simulink model "StewartDynamics"  (R2015a)
settings: Solver=ode45  StartTime=0.0  StopTime=10.0  RelTol=1e-3
undefined symbols (not defined in the file or in its folder): body_pts
libraries: simulink x1
settings Model: Creator=admin  LastModifiedBy=admin

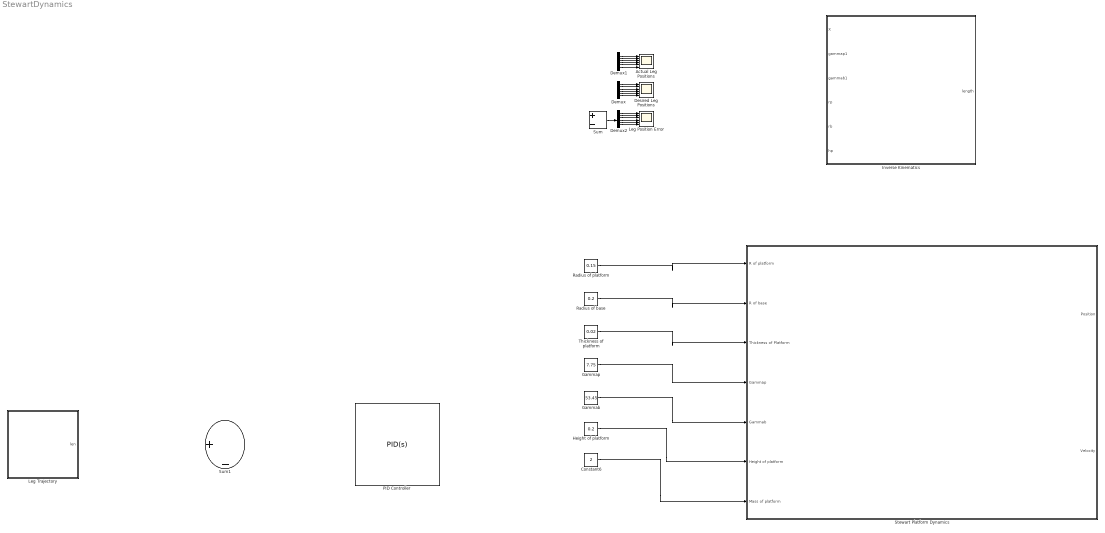
== system StewartDynamics ==
  Actual Leg Positions : Scope  NumInputPorts=6
      settings: TimeRange=10  YMin=0~1~0~0~0~0  YMax=14~14~13~14~13~13  SaveName=ScopeData5
  Constant6 : Constant  Value=2
  Demux : Demux  Outputs=6
  Demux1 : Demux  Outputs=6
  Demux2 : Demux  Outputs=6
  Desired Leg Positions : Scope  NumInputPorts=6
      settings: YMin=0~0~0~0~0~0  YMax=15~15~13~13~14~14  SaveName=ScopeData4
  Gammab : Constant  Value=53.45
  Gammap : Constant  Value=7.75
  Height of platform : Constant  Value=0.2
  Inverse Kinematics : MATLAB Function  TreatAsAtomicUnit=on
  Leg Trajectory : Subsystem
  Leg Position Error : Scope  NumInputPorts=6
      settings: YMin=-0.2~-0.2~-0.2~-0.2~-0.2~-0.2  YMax=0.2~0.2~0.2~0.2~0.2~0.2  SaveName=ScopeData6
  PID Controller : simulink/Continuous/PID Controller  Controller=PID  TimeDomain=Continuous-time  SampleTime=-1  IntegratorMethod=Forward Euler  FilterMethod=Forward Euler  Form=Parallel  UseFilter=on  ControllerParametersSource=internal  P=1  I=1  D=0  N=100  InitialConditionSource=internal  InitialConditionForIntegrator=0  InitialConditionForFilter=0  ExternalReset=none  LimitOutput=off  UpperSaturationLimit=inf  LowerSaturationLimit=-inf  LinearizeAsGain=on  AntiWindupMode=none  Kb=1  TrackingMode=off  Kt=1  PParamMin=[]  PParamMax=[]  IParamMin=[]  IParamMax=[]  DParamMin=[]  DParamMax=[]  NParamMin=[]  NParamMax=[]  KbParamMin=[]  KbParamMax=[]  KtParamMin=[]  KtParamMax=[]  POutMin=[]  POutMax=[]  IOutMin=[]  IOutMax=[]  DOutMin=[]  DOutMax=[]  NOutMin=[]  NOutMax=[]  KbOutMin=[]  KbOutMax=[]  KtOutMin=[]  KtOutMax=[]  IntegratorOutMin=[]  IntegratorOutMax=[]  FilterOutMin=[]  FilterOutMax=[]  SumOutMin=[]  SumOutMax=[]  SumI1OutMin=[]  SumI1OutMax=[]  SumI2OutMin=[]  SumI2OutMax=[]  SumI3OutMin=[]  SumI3OutMax=[]  SumDOutMin=[]  SumDOutMax=[]  SaturationOutMin=[]  SaturationOutMax=[]  IntegratorContinuousStateAttributes=''  IntegratorStateMustResolveToSignalObject=off  IntegratorRTWStateStorageClass=Auto  FilterContinuousStateAttributes=''  FilterStateMustResolveToSignalObject=off  FilterRTWStateStorageClass=Auto  DifferentiatorICPrevScaledInput=0  DifferentiatorOutMin=[]  DifferentiatorOutMax=[]
  Radius of base : Constant  Value=0.2
  Radius of platform : Constant  Value=0.15
  Stewart Platform Dynamics : Subsystem
  Sum : Sum  Inputs=+-
  Sum1 : Sum  Inputs=|+-
  Thickness of platform : Constant  Value=0.02
  wires:
  Gammap/1 -> Stewart Platform Dynamics/4(Gammap)
  Gammab/1 -> Stewart Platform Dynamics/5(Gammab)
  Height of platform/1 -> Stewart Platform Dynamics/6("Height of platform ")
  Constant6/1 -> Stewart Platform Dynamics/7(Mass of platform)
  Demux/1 -> Desired Leg Positions/1
  Demux/2 -> Desired Leg Positions/2
  Demux/3 -> Desired Leg Positions/3
  Demux/4 -> Desired Leg Positions/4
  Demux/5 -> Desired Leg Positions/5
  Demux/6 -> Desired Leg Positions/6
  Demux1/1 -> Actual Leg Positions/1
  Demux1/2 -> Actual Leg Positions/2
  Demux1/3 -> Actual Leg Positions/3
  Demux1/4 -> Actual Leg Positions/4
  Demux1/5 -> Actual Leg Positions/5
  Demux1/6 -> Actual Leg Positions/6
  Demux2/1 -> Leg Position Error/1
  Demux2/2 -> Leg Position Error/2
  Demux2/3 -> Leg Position Error/3
  Demux2/4 -> Leg Position Error/4
  Demux2/5 -> Leg Position Error/5
  Demux2/6 -> Leg Position Error/6
  Sum/1 -> Demux2/1
  Radius of platform/1 -> Stewart Platform Dynamics/1(R of platform)
  Radius of base/1 -> Stewart Platform Dynamics/2(R of base)
  Thickness of platform/1 -> Stewart Platform Dynamics/3(Thickness of Platform)
  ? -> ?
  ? -> ?
  ? -> ?
  ? -> ?

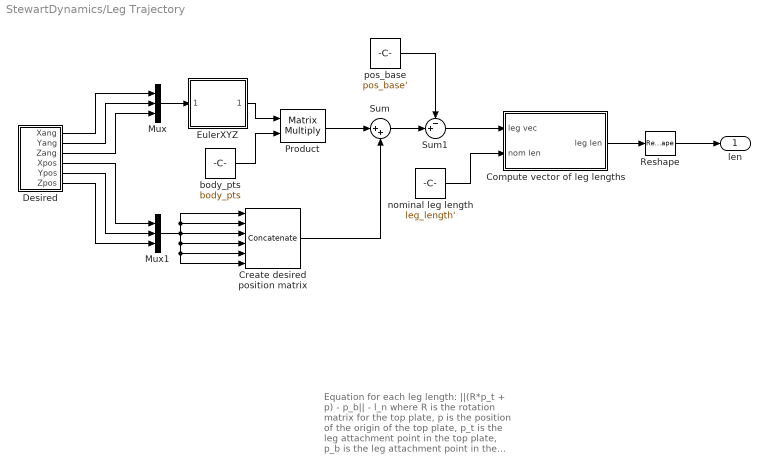
== system StewartDynamics/Leg Trajectory ==
  note: Equation for each leg length:
      | ||(R*p_t + p) - p_b|| - l_n
      | where R is the rotation matrix
      | for the top plate, p is the position
      | of the origin of the top plate, p_t
      | is the leg attachment point in the
      | top plate, p_b is the leg attachment
      | point in the base, and l_n is the
      | nominal distance between the
      | top and base attachment points.
  Compute vector of leg lengths : Subsystem  TreatAsAtomicUnit=on
  Create desired position matrix : Concatenate  NumInputs=6  Mode=Multidimensional array  ConcatenateDimension=2
  Desired : Subsystem
  EulerXYZ : Subsystem  AncestorBlock=|  mask(EulerXYZ){}
      | aerospace/Axes
      | Transformations/Direction Cosine Matrix
      | from Euler Angles
      mask help: Creates the EulerXYZ rotation matrix corresponding to body fixed rotations in the X, Y, and then Z. This matrix maps body vectors to world vectors.
      mask Help:
      | <p>This block determines the EulerXYZ matrix from a 3x1 euler angles in the X, Y, & Z directions. The matrix maps vectors the body axes to the inertial axes.</p>
      | 
      | <p>The block input and output contain more than one signal as described below.</p>
      | 
      | <p><H4>Block Vector Input - Euler XYZ angles</H4>
      |     <ul>
      |     <li>X angle</li>
      |     <li>Y angle</li>
      |     <li>Z angle</li>
      |    </ul>
      |    </p>
      | 
      | <p><H4>Block Matrix Output - XYZ Euler Matrix </H4>
      |     <ul>
      |    </ul>
      |    </p>
      mask Display: disp('Rotation\nMatrix')
  Mux : Mux  Inputs=3
  Mux1 : Mux  Inputs=3
  Product : Product  Multiplication=Matrix(*)  SaturateOnIntegerOverflow=on  InputSameDT=on  OutDataTypeStr=Inherit: Same as first input
  Reshape : Reshape
  Sum : Sum  Inputs=|++  SaturateOnIntegerOverflow=on  InputSameDT=on  OutDataTypeStr=Inherit: Same as first input
  Sum1 : Sum  Inputs=-+|  SaturateOnIntegerOverflow=on  InputSameDT=on  OutDataTypeStr=Inherit: Same as first input
  body_pts : Constant  Value=body_pts  VectorParams1D=off
  nominal leg length : Constant  Value=leg_length'  VectorParams1D=off
  pos_base : Constant  Value=pos_base'  VectorParams1D=off
  len : Outport
  wires:
  Mux/1 -> EulerXYZ/1(x y z angles)
  EulerXYZ/1(EulerXYZ) -> Product/1
  body_pts/1 -> Product/2
  Product/1 -> Sum/1
  Mux1/1 -> Create desired position matrix/1, Create desired position matrix/2, Create desired position matrix/4, Create desired position matrix/5, Create desired position matrix/6, Create desired position matrix/3
  Create desired position matrix/1 -> Sum/2
  pos_base/1 -> Sum1/1
  Sum/1 -> Sum1/2
  Sum1/1 -> Compute vector of leg lengths/1(leg vec)
  nominal leg length/1 -> Compute vector of leg lengths/2(nom len)
  Compute vector of leg lengths/1(leg len) -> Reshape/1
  Desired/3(Zang) -> Mux/3
  Desired/1(Xang) -> Mux/1
  Desired/2(Yang) -> Mux/2
  Desired/4(Xpos) -> Mux1/1
  Desired/5(Ypos) -> Mux1/2
  Desired/6(Zpos) -> Mux1/3
  Reshape/1 -> len/1

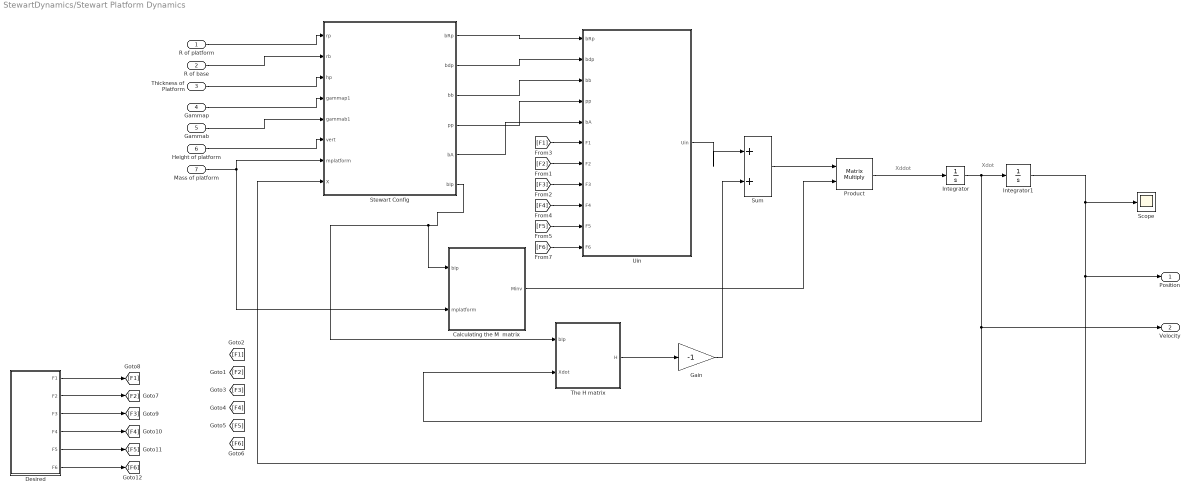
== system StewartDynamics/Stewart Platform Dynamics ==
  note: Xdot
  note: Xddot
  R of platform : Inport
  R of base : Inport  Port=2
  Thickness of Platform : Inport  Port=3
  Gammap : Inport  Port=4
  Gammab : Inport  Port=5
  "Height of platform " : Inport  Port=6
  Mass of platform : Inport  Port=7
  Calculating the M  matrix : MATLAB Function  TreatAsAtomicUnit=on
  Desired : Subsystem
  Gain : Gain  Gain=-1
  Integrator : Integrator
  Integrator1 : Integrator
  Product : Product  Multiplication=Matrix(*)
  Scope : Scope
  Stewart Config : MATLAB Function  TreatAsAtomicUnit=on
  Sum : Sum  Inputs=|++
  The H matrix : MATLAB Function  TreatAsAtomicUnit=on
  Uin : MATLAB Function  TreatAsAtomicUnit=on
  Position : Outport
  Velocity : Outport  Port=2
  wires:
  R of platform/1 -> Stewart Config/1(rp)
  "Height of platform "/1 -> Stewart Config/6(vert)
  Gammap/1 -> Stewart Config/4(gammap1)
  Gammab/1 -> Stewart Config/5(gammab1)
  Thickness of Platform/1 -> Stewart Config/3(hp)
  Mass of platform/1 -> Calculating the M  matrix/2(mplatform), Stewart Config/7(mplatform)
  R of base/1 -> Stewart Config/2(rb)
  Stewart Config/6(bIp) -> Calculating the M  matrix/1(bIp), The H matrix/1(bIp)
  Stewart Config/5(bA) -> Uin/5(bA)
  Stewart Config/4(pp) -> Uin/4(pp)
  Integrator1/1 -> Scope/1, Position/1, Stewart Config/8(X)
  Integrator/1 -> Integrator1/1, Velocity/1, The H matrix/2(Xdot)
  Product/1 -> Integrator/1
  The H matrix/1(H) -> Gain/1
  Stewart Config/1(bRp) -> Uin/1(bRp)
  Calculating the M  matrix/1(Minv) -> Product/2
  Sum/1 -> Product/1
  Stewart Config/3(bb) -> Uin/3(bb)
  Uin/1(Uin) -> Sum/1
  Stewart Config/2(bdp) -> Uin/2(bdp)
  Gain/1 -> Sum/2
  ? -> [F1]
  ? -> [F2]
  ? -> [F3]
  ? -> [F4]
  ? -> [F5]
  ? -> [F6]
  [F1] -> Uin/6(F1)
  [F2] -> Uin/7(F2)
  [F3] -> Uin/8(F3)
  [F4] -> Uin/9(F4)
  [F5] -> Uin/10(F5)
  [F6] -> Uin/11(F6)
  Desired/1(F1) -> [F1]
  Desired/2(F2) -> [F2]
  Desired/3(F3) -> [F3]
  Desired/4(F4) -> [F4]
  Desired/5(F5) -> [F5]
  Desired/6(F6) -> [F6]

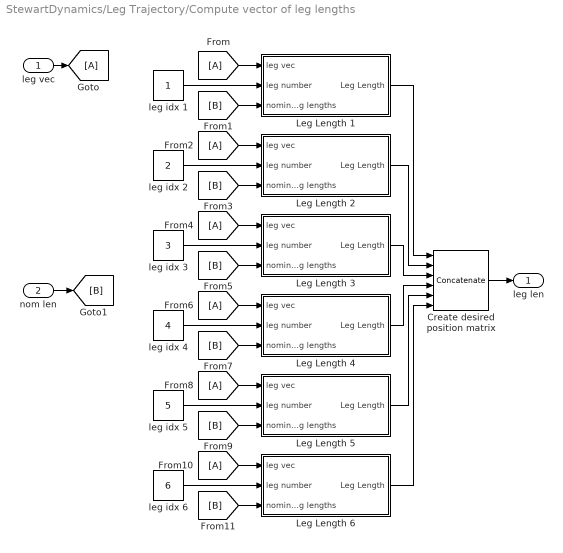
== system StewartDynamics/Leg Trajectory/Compute vector of leg lengths ==
  leg vec : Inport
  nom len : Inport  Port=2
  Create desired position matrix : Concatenate  NumInputs=6  Mode=Multidimensional array  ConcatenateDimension=2
  Leg Length 1 : Subsystem
  Leg Length 2 : Subsystem
  Leg Length 3 : Subsystem
  Leg Length 4 : Subsystem
  Leg Length 5 : Subsystem
  Leg Length 6 : Subsystem
  leg idx 1 : Constant
  leg idx 2 : Constant  Value=2
  leg idx 3 : Constant  Value=3
  leg idx 4 : Constant  Value=4
  leg idx 5 : Constant  Value=5
  leg idx 6 : Constant  Value=6
  leg len : Outport
  wires:
  Leg Length 6/1(Leg Length) -> Create desired position matrix/6
  Leg Length 5/1(Leg Length) -> Create desired position matrix/5
  Leg Length 4/1(Leg Length) -> Create desired position matrix/4
  Leg Length 3/1(Leg Length) -> Create desired position matrix/3
  Leg Length 2/1(Leg Length) -> Create desired position matrix/2
  Leg Length 1/1(Leg Length) -> Create desired position matrix/1
  [B] -> Leg Length 6/3(nominal leg lengths)
  [A] -> Leg Length 6/1(leg vec)
  leg idx 6/1 -> Leg Length 6/2(leg number)
  [B] -> Leg Length 5/3(nominal leg lengths)
  [A] -> Leg Length 5/1(leg vec)
  leg idx 5/1 -> Leg Length 5/2(leg number)
  [B] -> Leg Length 4/3(nominal leg lengths)
  [A] -> Leg Length 4/1(leg vec)
  leg idx 4/1 -> Leg Length 4/2(leg number)
  [B] -> Leg Length 3/3(nominal leg lengths)
  [A] -> Leg Length 3/1(leg vec)
  leg idx 3/1 -> Leg Length 3/2(leg number)
  [B] -> Leg Length 2/3(nominal leg lengths)
  [A] -> Leg Length 2/1(leg vec)
  leg idx 2/1 -> Leg Length 2/2(leg number)
  [B] -> Leg Length 1/3(nominal leg lengths)
  nom len/1 -> [B]
  [A] -> Leg Length 1/1(leg vec)
  leg vec/1 -> [A]
  leg idx 1/1 -> Leg Length 1/2(leg number)
  Create desired position matrix/1 -> leg len/1

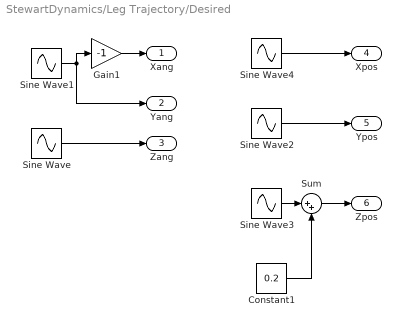
== system StewartDynamics/Leg Trajectory/Desired ==
  Constant1 : Constant  Value=0.2
  Gain1 : Gain  Gain=-1  SaturateOnIntegerOverflow=on  OutDataTypeStr=Inherit: Same as input  ParamDataTypeStr=Inherit: Same as input
  Sine Wave : Sin  Amplitude=0.03  Frequency=3  SampleTime=0
  Sine Wave1 : Sin  Amplitude=0.03  Frequency=3  SampleTime=0
  Sine Wave2 : Sin  Amplitude=0.025  Frequency=3  Phase=pi/2  SampleTime=0
  Sine Wave3 : Sin  Amplitude=0.025  Frequency=3  SampleTime=0
  Sine Wave4 : Sin  Amplitude=0.035  Frequency=3  SampleTime=0
  Sum : Sum  Inputs=|++  SaturateOnIntegerOverflow=on  InputSameDT=on  OutDataTypeStr=Inherit: Same as first input
  Xang : Outport
  Yang : Outport  Port=2
  Zang : Outport  Port=3
  Xpos : Outport  Port=4
  Ypos : Outport  Port=5
  Zpos : Outport  Port=6
  wires:
  Sine Wave/1 -> Zang/1
  Sine Wave1/1 -> Yang/1, Gain1/1
  Gain1/1 -> Xang/1
  Sine Wave2/1 -> Ypos/1
  Sine Wave3/1 -> Sum/1
  Sum/1 -> Zpos/1
  Constant1/1 -> Sum/2
  Sine Wave4/1 -> Xpos/1

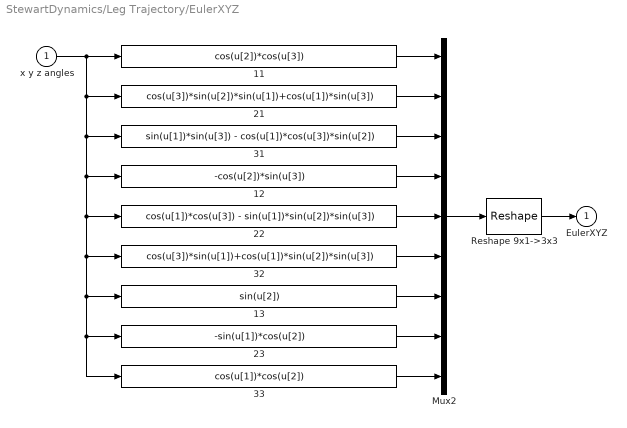
== system StewartDynamics/Leg Trajectory/EulerXYZ ==
  x y z angles : Inport
  11 : Fcn  Expr=cos(u[2])*cos(u[3])
  12 : Fcn  Expr=-cos(u[2])*sin(u[3])
  13 : Fcn  Expr=sin(u[2])
  21 : Fcn  Expr=cos(u[3])*sin(u[2])*sin(u[1])+cos(u[1])*sin(u[3])
  22 : Fcn  Expr=cos(u[1])*cos(u[3]) - sin(u[1])*sin(u[2])*sin(u[3])
  23 : Fcn  Expr=-sin(u[1])*cos(u[2])
  31 : Fcn  Expr=sin(u[1])*sin(u[3]) - cos(u[1])*cos(u[3])*sin(u[2])
  32 : Fcn  Expr=cos(u[3])*sin(u[1])+cos(u[1])*sin(u[2])*sin(u[3])
  33 : Fcn  Expr=cos(u[1])*cos(u[2])
  Mux2 : Mux  Inputs=9
  Reshape 9x1->3x3 : Reshape  OutputDimensionality=Customize  OutputDimensions=[3,3]
  EulerXYZ : Outport  InitialOutput=0
  wires:
  x y z angles/1 -> 23/1, 33/1, 13/1, 32/1, 22/1, 12/1, 31/1, 21/1, 11/1
  33/1 -> Mux2/9
  23/1 -> Mux2/8
  13/1 -> Mux2/7
  32/1 -> Mux2/6
  22/1 -> Mux2/5
  12/1 -> Mux2/4
  31/1 -> Mux2/3
  21/1 -> Mux2/2
  11/1 -> Mux2/1
  Mux2/1 -> Reshape 9x1->3x3/1
  Reshape 9x1->3x3/1 -> EulerXYZ/1

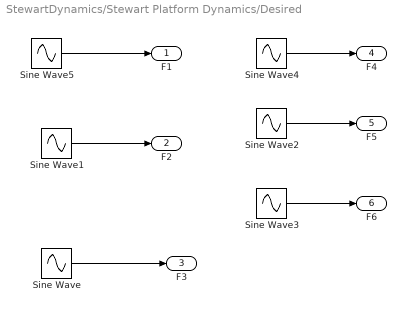
== system StewartDynamics/Stewart Platform Dynamics/Desired ==
  Sine Wave : Sin  Amplitude=0.29  Frequency=0.6283  SampleTime=0
  Sine Wave1 : Sin  Amplitude=0.3  Frequency=0.628  Phase=1.57  SampleTime=0
  Sine Wave2 : Sin  Amplitude=0.305  Frequency=0.6283  SampleTime=0
  Sine Wave3 : Sin  Amplitude=0.28  Frequency=0.6283  Phase=1.57  SampleTime=0
  Sine Wave4 : Sin  Amplitude=0.31  Frequency=0.6283  Phase=1.57  SampleTime=0
  Sine Wave5 : Sin  Amplitude=0.3  Frequency=0.628  SampleTime=0
  F1 : Outport
  F2 : Outport  Port=2
  F3 : Outport  Port=3
  F4 : Outport  Port=4
  F5 : Outport  Port=5
  F6 : Outport  Port=6
  wires:
  Sine Wave/1 -> F3/1
  Sine Wave1/1 -> F2/1
  Sine Wave5/1 -> F1/1
  Sine Wave2/1 -> F5/1
  Sine Wave3/1 -> F6/1
  Sine Wave4/1 -> F4/1

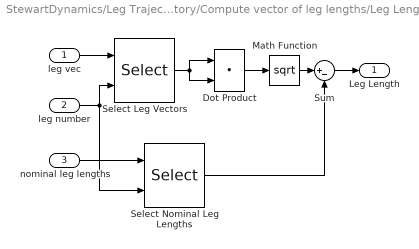
== system StewartDynamics/Leg Trajectory/Compute vector of leg lengths/Leg Length 1 ==
  leg vec : Inport
  leg number : Inport  Port=2
  nominal leg lengths : Inport  Port=3
  Dot Product : DotProduct  InputSameDT=on  OutDataTypeStr=Inherit: Inherit via internal rule
  Math Function : Math  Operator=sqrt  SaturateOnIntegerOverflow=on
  Select Leg Vectors : Selector  NumberOfDimensions=2  InputPortWidth=3  IndexOptions=Select all,Index vector (port)  Indices=-1,1
  Select Nominal Leg Lengths : Selector  InputPortWidth=6  IndexOptions=Index vector (port)  Indices=[1 3]
  Sum : Sum  Inputs=|+-  SaturateOnIntegerOverflow=on  InputSameDT=on  OutDataTypeStr=Inherit: Same as first input
  Leg Length : Outport
  wires:
  nominal leg lengths/1 -> Select Nominal Leg Lengths/1
  Sum/1 -> Leg Length/1
  leg vec/1 -> Select Leg Vectors/1
  leg number/1 -> Select Leg Vectors/2, Select Nominal Leg Lengths/2
  Dot Product/1 -> Math Function/1
  Select Leg Vectors/1 -> Dot Product/1, Dot Product/2
  Math Function/1 -> Sum/1
  Select Nominal Leg Lengths/1 -> Sum/2

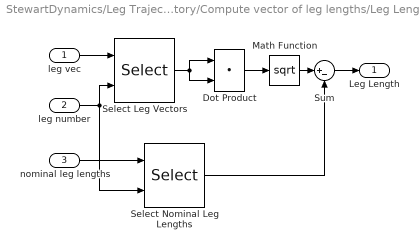
== system StewartDynamics/Leg Trajectory/Compute vector of leg lengths/Leg Length 2 ==
  leg vec : Inport
  leg number : Inport  Port=2
  nominal leg lengths : Inport  Port=3
  Dot Product : DotProduct  InputSameDT=on  OutDataTypeStr=Inherit: Inherit via internal rule
  Math Function : Math  Operator=sqrt  SaturateOnIntegerOverflow=on
  Select Leg Vectors : Selector  NumberOfDimensions=2  InputPortWidth=3  IndexOptions=Select all,Index vector (port)  Indices=-1,1
  Select Nominal Leg Lengths : Selector  InputPortWidth=6  IndexOptions=Index vector (port)  Indices=[1 3]
  Sum : Sum  Inputs=|+-  SaturateOnIntegerOverflow=on  InputSameDT=on  OutDataTypeStr=Inherit: Same as first input
  Leg Length : Outport
  wires:
  nominal leg lengths/1 -> Select Nominal Leg Lengths/1
  Sum/1 -> Leg Length/1
  leg vec/1 -> Select Leg Vectors/1
  leg number/1 -> Select Leg Vectors/2, Select Nominal Leg Lengths/2
  Dot Product/1 -> Math Function/1
  Select Leg Vectors/1 -> Dot Product/1, Dot Product/2
  Math Function/1 -> Sum/1
  Select Nominal Leg Lengths/1 -> Sum/2

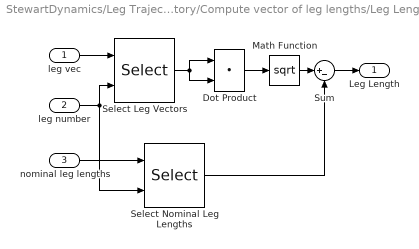
== system StewartDynamics/Leg Trajectory/Compute vector of leg lengths/Leg Length 3 ==
  leg vec : Inport
  leg number : Inport  Port=2
  nominal leg lengths : Inport  Port=3
  Dot Product : DotProduct  InputSameDT=on  OutDataTypeStr=Inherit: Inherit via internal rule
  Math Function : Math  Operator=sqrt  SaturateOnIntegerOverflow=on
  Select Leg Vectors : Selector  NumberOfDimensions=2  InputPortWidth=3  IndexOptions=Select all,Index vector (port)  Indices=-1,1
  Select Nominal Leg Lengths : Selector  InputPortWidth=6  IndexOptions=Index vector (port)  Indices=[1 3]
  Sum : Sum  Inputs=|+-  SaturateOnIntegerOverflow=on  InputSameDT=on  OutDataTypeStr=Inherit: Same as first input
  Leg Length : Outport
  wires:
  nominal leg lengths/1 -> Select Nominal Leg Lengths/1
  Sum/1 -> Leg Length/1
  leg vec/1 -> Select Leg Vectors/1
  leg number/1 -> Select Leg Vectors/2, Select Nominal Leg Lengths/2
  Dot Product/1 -> Math Function/1
  Select Leg Vectors/1 -> Dot Product/1, Dot Product/2
  Math Function/1 -> Sum/1
  Select Nominal Leg Lengths/1 -> Sum/2

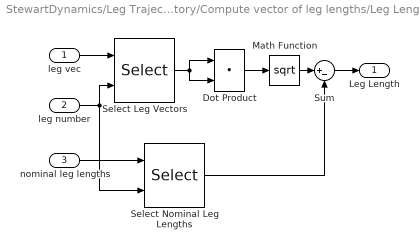
== system StewartDynamics/Leg Trajectory/Compute vector of leg lengths/Leg Length 4 ==
  leg vec : Inport
  leg number : Inport  Port=2
  nominal leg lengths : Inport  Port=3
  Dot Product : DotProduct  InputSameDT=on  OutDataTypeStr=Inherit: Inherit via internal rule
  Math Function : Math  Operator=sqrt  SaturateOnIntegerOverflow=on
  Select Leg Vectors : Selector  NumberOfDimensions=2  InputPortWidth=3  IndexOptions=Select all,Index vector (port)  Indices=-1,1
  Select Nominal Leg Lengths : Selector  InputPortWidth=6  IndexOptions=Index vector (port)  Indices=[1 3]
  Sum : Sum  Inputs=|+-  SaturateOnIntegerOverflow=on  InputSameDT=on  OutDataTypeStr=Inherit: Same as first input
  Leg Length : Outport
  wires:
  nominal leg lengths/1 -> Select Nominal Leg Lengths/1
  Sum/1 -> Leg Length/1
  leg vec/1 -> Select Leg Vectors/1
  leg number/1 -> Select Leg Vectors/2, Select Nominal Leg Lengths/2
  Dot Product/1 -> Math Function/1
  Select Leg Vectors/1 -> Dot Product/1, Dot Product/2
  Math Function/1 -> Sum/1
  Select Nominal Leg Lengths/1 -> Sum/2

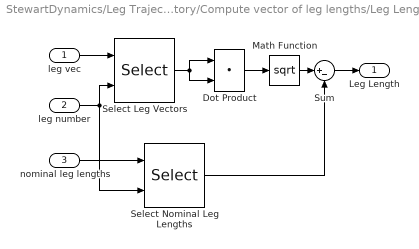
== system StewartDynamics/Leg Trajectory/Compute vector of leg lengths/Leg Length 5 ==
  leg vec : Inport
  leg number : Inport  Port=2
  nominal leg lengths : Inport  Port=3
  Dot Product : DotProduct  InputSameDT=on  OutDataTypeStr=Inherit: Inherit via internal rule
  Math Function : Math  Operator=sqrt  SaturateOnIntegerOverflow=on
  Select Leg Vectors : Selector  NumberOfDimensions=2  InputPortWidth=3  IndexOptions=Select all,Index vector (port)  Indices=-1,1
  Select Nominal Leg Lengths : Selector  InputPortWidth=6  IndexOptions=Index vector (port)  Indices=[1 3]
  Sum : Sum  Inputs=|+-  SaturateOnIntegerOverflow=on  InputSameDT=on  OutDataTypeStr=Inherit: Same as first input
  Leg Length : Outport
  wires:
  nominal leg lengths/1 -> Select Nominal Leg Lengths/1
  Sum/1 -> Leg Length/1
  leg vec/1 -> Select Leg Vectors/1
  leg number/1 -> Select Leg Vectors/2, Select Nominal Leg Lengths/2
  Dot Product/1 -> Math Function/1
  Select Leg Vectors/1 -> Dot Product/1, Dot Product/2
  Math Function/1 -> Sum/1
  Select Nominal Leg Lengths/1 -> Sum/2

== system StewartDynamics/Leg Trajectory/Compute vector of leg lengths/Leg Length 6 ==
  leg vec : Inport
  leg number : Inport  Port=2
  nominal leg lengths : Inport  Port=3
  Dot Product : DotProduct  InputSameDT=on  OutDataTypeStr=Inherit: Inherit via internal rule
  Math Function : Math  Operator=sqrt  SaturateOnIntegerOverflow=on
  Select Leg Vectors : Selector  NumberOfDimensions=2  InputPortWidth=3  IndexOptions=Select all,Index vector (port)  Indices=-1,1
  Select Nominal Leg Lengths : Selector  InputPortWidth=6  IndexOptions=Index vector (port)  Indices=[1 3]
  Sum : Sum  Inputs=|+-  SaturateOnIntegerOverflow=on  InputSameDT=on  OutDataTypeStr=Inherit: Same as first input
  Leg Length : Outport
  wires:
  nominal leg lengths/1 -> Select Nominal Leg Lengths/1
  Sum/1 -> Leg Length/1
  leg vec/1 -> Select Leg Vectors/1
  leg number/1 -> Select Leg Vectors/2, Select Nominal Leg Lengths/2
  Dot Product/1 -> Math Function/1
  Select Leg Vectors/1 -> Dot Product/1, Dot Product/2
  Math Function/1 -> Sum/1
  Select Nominal Leg Lengths/1 -> Sum/2

== matlab function StewartDynamics/Stewart Platform Dynamics/Stewart Config ==
  data: rp input; bRp output; rb input; hp input; gammap1 input; gammab1 input; vert input; mplatform input; X input; bdp output; bb output; pp output; bA output; bIp output
function [bRp,bdp,bb,pp,bA,bIp] = fcn(rp,rb,hp,gammap1,gammab1,vert,mplatform,X)
%#codegen
%The states that were chosen were X=[x,y,z,phi,theta,psi] and
%X2=[xdot,ydot,zdot,p,q,r ]
%Due to this a  trnasformation matrix must be added to transform the body
%rates to Euler rates.
gammap = [gammap1,120-gammap1, 120+gammap1, -120-gammap1,-120+gammap1,-gammap1];
gammab = [gammab1,120-gammab1, 120+gammab1, -120-gammab1,-120+gammab1,-gammab1];

 %alphap = [0 , 120, 120, -120 , -120 , 0] ;  
 %betab = [60,60,180,180,-60,-60];
 
 
 % pIp = mplatform *[((rp^2)/4) , 0, 0; 0, ((rp*2)/4), 0; 0, 0, (rp^2)/2] ;
    pp=zeros(3,6);
    pp(1,: ) = rp*cos(gammap*pi/180);
    pp(2,: ) = rp*sin(gammap*pi/180) ;
    pp(3,: ) = [hp/2,hp/2,hp/2,hp/2,hp/2,hp/2 ] ;        %hp is the thickness of the platform
    bb=zeros(3,6);
    bb(1,: ) = rb*cos(gammab*pi/180);
    bb(2,: ) = rb*sin(gammab*pi/180);
    bb(3,: ) = [0 , 0, 0, 0 , 0, 0] ;
    
     bdp = [X(1,a),X(2,a),X(3,a)+vert]' ;                        %Position of platform frame wrt base
    bDp = [bdp,bdp,bdp,bdp,bdp,bdp] ;                           %This is same for all 6 actuators
   
      psi=X(4,a);
      the=X(5,a);
      phi=X(6,a);
    
   
    spsi = sin(psi);
    cpsi = cos(psi);
    sthe = sin(the);
    cthe = cos(the);
    sphi = sin(phi);
    cphi = cos(phi);
    
    
    pIp = mplatform *[((0.15^2)/4) , 0, 0; 0, ((0.15*2)/4), 0; 0, 0, (0.15^2)/2] ;
    bRp=zeros(3,3);
    bRp(1,1 ) = cphi * cthe ;
    bRp(1,2 ) = -sphi*cpsi + cphi * sthe * spsi ;
    bRp(1,3 ) = sphi * spsi + cphi * sthe * cpsi ;
    bRp(2,1 ) = sphi * cthe ;
    bRp(2,2 ) = cphi * cpsi + sphi * sthe * spsi ;
    bRp(2,3 ) = -cphi * spsi + sphi * sthe * cpsi ;
    bRp(3,1 ) = -sthe ;
    bRp(3,2 ) = cthe * spsi ;
    bRp(3,3 ) = cthe * cpsi ;
    
     bA = bRp*pp + bDp - bb ;                                    %Actuator vector
    
     bIp=bRp*pIp*bRp';                                           %Inertia tensor varying due to orientation of platform wrt base

== matlab function StewartDynamics/Inverse Kinematics ==
  data: X input; length output; gammap1 input; gammab1 input; rp input; rb input; hp input
function length = fcn(X,gammap1,gammab1,rp,rb,hp)
%#codegen
%Define the system parameters


gammap = [gammap1,120-gammap1, 120+gammap1, -120-gammap1,-120+gammap1,-gammap1];

%gammabl = 21.1495 ; % unit in degree
gammab = [gammab1,120-gammab1, 120+gammab1, -120-gammab1,-120+gammab1,-gammab1];

x=X(1,1);
y=X(2,1);
z=X(3,1);
psi=X(4,1);
the=X(5,1);
phi=X(6,1);

spsi = sin(psi*pi/180 );
cpsi = cos(psi*pi/180 );
sthe = sin(the*pi/180 );
cthe = cos(the*pi/180 );
sphi = sin(phi*pi/180 );
cphi = cos(phi*pi/180 );
bRp=zeros(3,3);

% rotation matrix R
bRp(1,1 ) = cphi * cthe ;
bRp(1,2 ) = -sphi * cpsi + cphi * sthe * spsi ;
bRp(1,3 ) = sphi * spsi + cphi * sthe * cpsi ;
bRp(2,1 ) = sphi * cthe ;
bRp(2,2 ) = cphi * cpsi + sphi * sthe * spsi ;
bRp(2,3 ) = -cphi * spsi + sphi * sthe * cpsi ;
bRp(3,1 ) = -sthe ;
bRp(3,2 ) = cthe * spsi ;
bRp(3,3 ) = cthe * cpsi ;

% fixed vector of pp
pp=zeros(3,6);
pp(1,: ) = rp*cos(gammap*pi/180);
pp(2,: ) = rp*sin(gammap*pi/180) ;
pp(3,: ) = [hp/2,hp/2,hp/2,hp/2,hp/2,hp/2 ] ;

%fixed vector of bb
bb=zeros(3,6);
bb(1,: ) = rb*cos(gammab*pi/180);
bb(2,: ) = rb*sin(gammab*pi/180) ;
bb(3,: ) = [0,0,0,0,0,0] ;
% bdp

bdp = [x,y,z ]' ;
bDp = [bdp,bdp,bdp,bdp,bdp,bdp] ;
% actuator vector
bA = bRp*pp +bDp - bb ;
length=zeros(6,1);
for i =1:6 
length(i,1) = norm(bA(:,i)) ;
end

== matlab function StewartDynamics/Stewart Platform Dynamics/Uin ==
  data: bRp input; bdp input; bb input; Uin output; pp input; bA input; F1 input; F2 input; F3 input; F4 input; F5 input; F6 input
function Uin = fcn(bRp,bdp,bb,pp,bA,F1,F2,F3,F4,F5,F6)
%#codegen
    g=9.81;
    G=[0,0,-g]';
    Fvec=zeros(3,6);
    %We are going to add g in vector form to the input force
   
    %for j=1:6
     %  Fvec(:,j)=F(j,a)*bA(:,j);
    %end
    Fvec(:,1)=F1*bA(:,1);
    Fvec(:,2)=F2*bA(:,2);
    Fvec(:,3)=F3*bA(:,3);
    Fvec(:,4)=F4*bA(:,4);
    Fvec(:,5)=F5*bA(:,5);
    Fvec(:,6)=F6*bA(:,6);
      
    
   U=zeros(6,1);                                              %Combined effect of gravity and force on actuators
     %for j=1:6
      % U(j,1)= F(j,a)+dot(Fvec(:,j),G);
     %end
     
     
     U(1,1)=F1+dot(Fvec(:,1),G);
     U(2,1)=F2+dot(Fvec(:,2),G);
     U(3,1)=F3+dot(Fvec(:,3),G);
     U(4,1)=F4+dot(Fvec(:,4),G);
     U(5,1)=F5+dot(Fvec(:,5),G);
     U(6,1)=F6+dot(Fvec(:,6),G);
    
     Jt=zeros(6,6);
   
      for i=1:6
      Jt(:,i ) = [ ( bRp*pp(:,i) + bdp - bb(:,i) ); cross( bRp*pp(:,i),bdp-bb(:,i) ) ] / norm(bA(:,i)) ;
  
      end
    
     Uin=Jt*U;                                                %Input u in state space form

== matlab function StewartDynamics/Stewart Platform Dynamics/Calculating the M  matrix ==
  data: bIp input; mplatform input; Minv output
function Minv = fcn(bIp,mplatform)
%#codegen

m=mplatform*(eye(3));

z=zeros(3,3);

M=[m,z;z,bIp];
Minv=inv(M);

== matlab function StewartDynamics/Stewart Platform Dynamics/The H matrix ==
  data: bIp input; H output; Xdot input
function H = fcn(bIp,Xdot)
%#codegen
bWp = [Xdot(4,1) ; Xdot(5,1) ; Xdot(6,1)] ;

bWpskew=[ 0 , -1*bWp(3,1) , bWp(2,1) ; 
         bWp(3,1) , 0 , -1*bWp(1,1)  ;
         -1*bWp(2,1), bWp(1,1), 0 ];
     
     h= bWpskew*bIp;                             %WxI 
    H=[z,z;z,h];
